simulink model "platform"  (R2019a)
settings: Solver=ode4  StartTime=0.0  StopTime=time_end  FixedStep=0.01  RelTol=1e-3  EnableMultiTasking=on
values from neighbouring files (symbols this model uses):
  A = [zeros(2*M,2*M) eye(2*M);zeros(2*M,2*M) l*eye(2*M)]    [main.m]    (also in mydistance.m = repmat(x,1,sz(2)) - S)
  B = [zeros(2*M,2*M);-l*eye(2*M)]    [main.m]
  C = eye(4*M)    [main.m]
  D = zeros(4*M,2*M)    [main.m]
  Initialcondition = [InitialPosition;zeros(2*M,1)]    [main.m]
  InitialPosition = [InitialPosition;UavTeam.Uav(k).CurrentPos]    [UAVInitialization.m]
  M = UavTeam.AvailableNumMax    [AttitudeDynamics.m]    (also in MyMap.m; MyMap_init.m; collisioncon.m; dangerdistance.m)
  UavTeam = UAVInitialization(M,rm,l,vmax)    [main.m]
settings Model: SimulationMode=accelerator  Creator=Furao  LastModifiedBy=Furao
settings DataIOCC: LimitDataPoints=on  SaveFormat=Array  ReturnWorkspaceOutputs=off  SignalLoggingName=sigsOut
settings DebuggingCC: SaveWithParameterizedLinksMsg=none  UnderspecifiedInitializationDetection=Classic  MergeDetectMultiDrivingBlocksExec=none  SignalResolutionControl=TryResolveAllWithWarning  MultiTaskDSMMsg=warning  MultiTaskCondExecSysMsg=none  ArithmeticOperatorsInVariantConditions=warning
settings HardwareCC: ProdBitPerPointer=32  ProdBitPerSizeT=32  ProdBitPerPtrDiffT=32  ProdLargestAtomicFloat=None  ProdIntDivRoundTo=Undefined  ProdEndianess=Unspecified  ProdWordSize=32  ProdHWDeviceType=32-bit Generic  TargetUnknown=on
settings ModelReferenceCC: PropagateSignalLabelsOutOfModel=off
settings SFSimCC: SimUseLocalCustomCode=off
settings RTWCC: RTWUseLocalCustomCode=off
settings CodeAppCC: StateflowObjectComments=on
settings GRTTargetCC: TargetLangStandard=C89/C90 (ANSI)  CombineOutputUpdateFcns=off  GRTInterface=on
settings ConfigComp: CovMetricSettings=dw  CovHtmlReporting=on  CovSaveCumulativeToWorkspaceVar=on  CovSaveSingleToWorkspaceVar=on  CovExternalEMLEnable=off

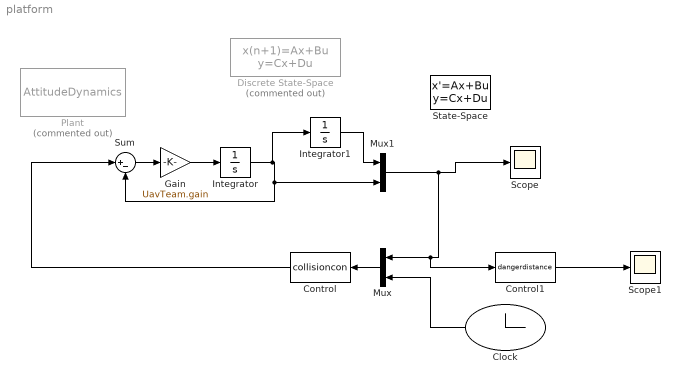
== system platform ==
  Clock : Clock
  Control : MATLABFcn  MATLABFcn=collisioncon
  Control1 : MATLABFcn  MATLABFcn=dangerdistance
  Discrete State-Space : DiscreteStateSpace  Commented=on  A=A  B=B  C=C  D=D  InitialCondition=Initialcondition  SampleTime=-1
  Gain : Gain  Gain=UavTeam.gain
  Integrator : Integrator  InitialCondition=zeros(2*M,1)
  Integrator1 : Integrator  InitialCondition=InitialPosition
  Mux : Mux  Inputs=2
  Mux1 : Mux  Inputs=2
  Plant : S-Function  Commented=on  FunctionName=AttitudeDynamics  SFunctionDeploymentMode=off  EnableBusSupport=off
  Scope : Scope
  Scope1 : Scope
  State-Space : StateSpace  A=A  B=B  C=C  D=D  InitialCondition=Initialcondition
  Sum : Sum  Inputs=|+-
  wires:
  Control1/1 -> Scope1/1
  Mux/1 -> Control/1
  Clock/1 -> Mux/2
  Control/1 -> Sum/1
  Sum/1 -> Gain/1
  Gain/1 -> Integrator/1
  Mux1/1 -> Control1/1, Mux/1, Scope/1
  Integrator1/1 -> Mux1/1
  Integrator/1 -> Mux1/2, Sum/2, Integrator1/1
